simulink model "filtro3_iir_sim_r2015a"  (Simulink 8.5)
settings: Solver=FixedStepDiscrete  SolverMode=SingleTasking  StartTime=0.0  StopTime=1  RelTol=1e-3
values from neighbouring files (symbols this model uses):
  fa = 10000    [filtro3_comparativo.m]    (also in filtro3_iir.m; filtro3_pm.m)
undefined symbols (not defined in the file or in its folder): Ta
libraries: dspsrcs4 x4, dsparch4 x2
settings Model: Creator=vini  LastModifiedBy=vini  CovMetricSettings=dwe  CovHtmlReporting=off  covSaveCumulativeToWorkspaceVar=off  CovSaveSingleToWorkspaceVar=off  CovExternalEMLEnable=on
settings DataIOCC: LimitDataPoints=off  SaveFormat=Dataset  SignalLoggingSaveFormat=Dataset
settings OptimizationCC: BlockReduction=off  ConditionallyExecuteInputs=off  InlineParams=on  ExpressionDepthLimit=128
settings DebuggingCC: AlgebraicLoopMsg=error  UnderspecifiedInitializationDetection=Simplified  MergeDetectMultiDrivingBlocksExec=error  FcnCallInpInsideContextMsg=EnableAllAsError  StateNameClashWarn=none  SFUnexpectedBacktrackingDiag=error  SFNoUnconditionalDefaultTransitionDiag=error
settings HardwareCC: ProdHWDeviceType=ASIC/FPGA->ASIC/FPGA  TargetBitPerLong=64  TargetBitPerPointer=64  TargetLongLongMode=on  TargetIntDivRoundTo=Zero  TargetEndianess=LittleEndian  TargetWordSize=64  TargetHWDeviceType=Custom Processor->MATLAB Host Computer  ProdEqTarget=off
settings ModelReferenceCC: PropagateSignalLabelsOutOfModel=on
settings SFSimCC: SimUseLocalCustomCode=on
settings RTWCC: RTWUseLocalCustomCode=on
settings GRTTargetCC: TargetLangStandard=C99 (ISO)  GeneratePreprocessorConditionals=Use local settings  CombineOutputUpdateFcns=on  GRTInterface=off

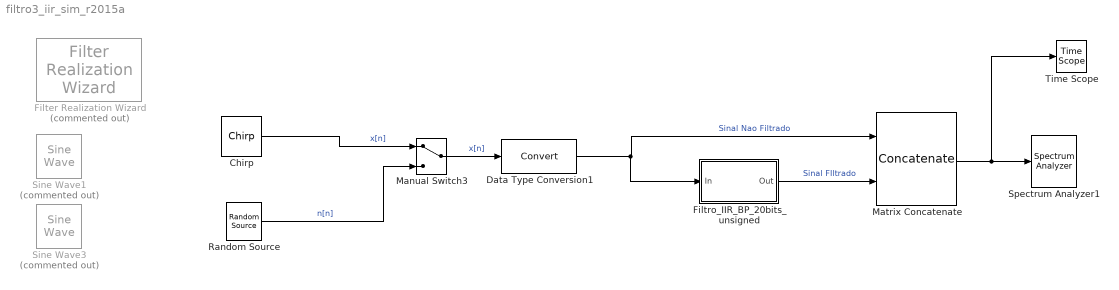
== system filtro3_iir_sim_r2015a ==
  Chirp : dspsrcs4/Chirp  sweep=Linear  mode=Unidirectional  f0=0  f1=fa/2  t1=1  Tsweep=1  phase=0  Ts=Ta  spf=spf  datatype=Double
  Data Type Conversion1 : DataTypeConversion
  Filter Realization Wizard : dsparch4/Filter Realization Wizard  Commented=on
  Filtro_IIR_BP_20bits_unsigned : Subsystem  Tag=BlockMethodSubSystem
  Manual Switch3 : ManualSwitch
  Matrix Concatenate : Concatenate  Mode=Multidimensional array  ConcatenateDimension=2
  Random Source : dspsrcs4/Random Source  SrcType=Uniform  NormMethod=Ziggurat  CltLength=12  MinVal=-1  MaxVal=1  MeanVal=0  VarVal=1  RepMode=Not repeatable  rawSeed=1  IsInherit=off  SampMode=Discrete  SampTime=Ta  SampFrame=spf  DataType=Single  OutComplex=Real
  Sine Wave1 : dspsrcs4/Sine Wave  Commented=on  Amplitude=1  Frequency=100  Phase=0  SampleMode=Discrete  OutComplex=Real  CompMethod=Trigonometric fcn  TableSize=Speed  SampleTime=1/8000  SamplesPerFrame=1  ResetState=Restart at time zero  dataType=double  wordLen=16  udDataType=sfix(16)  fracBitsMode=Best precision  numFracBits=15  OutDataTypeStr=double  LastOutDataTypeStr=double
  Sine Wave3 : dspsrcs4/Sine Wave  Commented=on  Amplitude=1  Frequency=100  Phase=0  SampleMode=Discrete  OutComplex=Real  CompMethod=Trigonometric fcn  TableSize=Speed  SampleTime=1/8000  SamplesPerFrame=1  ResetState=Restart at time zero  dataType=double  wordLen=16  udDataType=sfix(16)  fracBitsMode=Best precision  numFracBits=15  OutDataTypeStr=double  LastOutDataTypeStr=double
  Spectrum Analyzer1 : SpectrumAnalyzer
  Time Scope : TimeScope  DefaultConfigurationName=spbscopes.TimeScopeBlockCfg
  wires:
  Data Type Conversion1/1 -> Filtro_IIR_BP_20bits_unsigned/1(In), Matrix Concatenate/1  "Sinal Nao Filtrado"
  Matrix Concatenate/1 -> Time Scope/1, Spectrum Analyzer1/1
  Manual Switch3/1 -> Data Type Conversion1/1  "x[n]"
  Random Source/1 -> Manual Switch3/2  "n[n]"
  Chirp/1 -> Manual Switch3/1  "x[n]"
  Filtro_IIR_BP_20bits_unsigned/1(Out) -> Matrix Concatenate/2  "Sinal FIltrado"

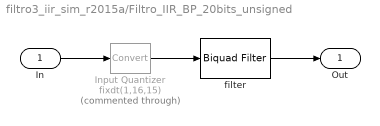
== system filtro3_iir_sim_r2015a/Filtro_IIR_BP_20bits_unsigned ==
  In : Inport
  Input Quantizer : DataTypeConversion  Commented=through  OutDataTypeStr=fixdt(1,16,15)  RndMeth=Round  SaturateOnIntegerOverflow=on
  filter : dsparch4/Biquad Filter  FilterSource=Specify via dialog  CoeffSource=Specify via dialog  FilterObject=BQF  IIRFiltStruct=Direct form II  BiQuadCoeffs=[1 0.353353948679126395 0.999999999999989342 1 0.814819011151262429 0.843633602697968277;1 1.40715579232338883 0.999999999999974687 1 0.965879710982947559 0.851011920331394722;1 0.725520024065602454 0.999999999999999445 1 0.812603367593793258 0.954924333743372933;1 1.17400488535383563 1.00000000000004086 1 1.0659691505063742 0.958842711800593106]  ScaleValues=[0.00853204727172851562;1;1;1;1]  IC=0  ICnum=0  ICden=0  a0Flag=Warning  optimizeScaleValues=on  ScaleValueMode=Specify via input port (g)  roundingMode=Convergent  overflowMode=off  stageInputMode=Binary point scaling  stageInputWordLength=16  stageInputFracLength=10  stageOutputMode=Binary point scaling  stageOutputWordLength=16  stageOutputFracLength=4  firstCoeffMode=Binary point scaling  firstCoeffWordLength=20  firstCoeffFracLength=19  scaleValueFracLength=26  prodOutputMode=Binary point scaling  prodOutputWordLength=36  prodOutputFracLength=26  denProdOutputFracLength=26  accumMode=Binary point scaling  accumWordLength=40  accumFracLength=26  denAccumFracLength=26  memoryMode=Binary point scaling  memoryWordLength=16  memoryFracLength=7  secondMemoryFracLength=15  outputMode=Binary point scaling  outputWordLength=16  outputFracLength=4
  Out : Outport
  wires:
  In/1 -> Input Quantizer/1
  Input Quantizer/1 -> filter/1
  filter/1 -> Out/1
